simulink model "PWM_Generator"  (R2025b)
settings: Solver=VariableStepAuto  StartTime=0.0  StopTime=0.15  RelTol=1e-3
libraries: simulink x1
settings Model: Creator=Sneha Shree K  LastModifiedBy=Sneha Shree K

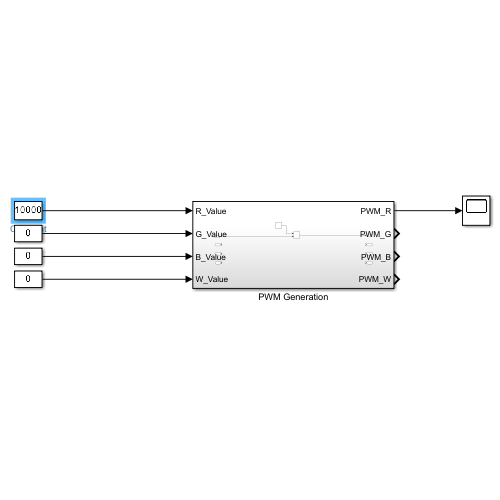
[thumbnail: Simulink's stored preview of the top-level diagram]
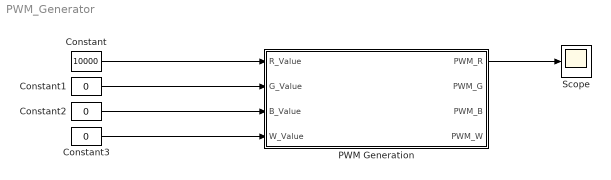
== system PWM_Generator ==
  Constant : Constant  Value=10000  OutDataTypeStr=uint16
  Constant1 : Constant  Value=0  OutDataTypeStr=uint16
  Constant2 : Constant  Value=0  OutDataTypeStr=uint16
  Constant3 : Constant  Value=0  OutDataTypeStr=uint16
  PWM Generation : Subsystem
  Scope : Scope
      settings: ActiveDisplayYMinimum=-0.12499999999999997  ActiveDisplayYMaximum=1.125
  wires:
  Constant/1 -> PWM Generation/1(R_Value)
  Constant1/1 -> PWM Generation/2(G_Value)
  Constant2/1 -> PWM Generation/3(B_Value)
  Constant3/1 -> PWM Generation/4(W_Value)
  PWM Generation/1(PWM_R) -> Scope/1

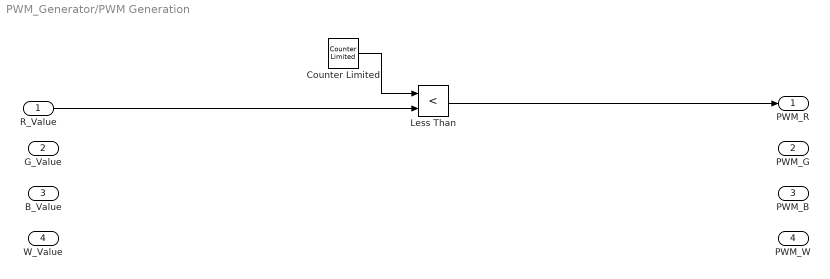
== system PWM_Generator/PWM Generation ==
  R_Value : Inport
  G_Value : Inport  Port=2
  B_Value : Inport  Port=3
  W_Value : Inport  Port=4
  Counter Limited : simulink/Sources/Counter Limited  uplimit=65535  tsamp=1e-6
  Less Than : RelationalOperator  Operator=<  OutDataTypeStr=boolean  RndMeth=Simplest  InputSameDT=off
  PWM_R : Outport
  PWM_G : Outport  Port=2
  PWM_B : Outport  Port=3
  PWM_W : Outport  Port=4
  wires:
  R_Value/1 -> Less Than/2
  Less Than/1 -> PWM_R/1
  Counter Limited/1 -> Less Than/1
